simulink model "qpsk_srrc"  (R2012b)
settings: Solver=ode45  StartTime=0.0  StopTime=10.0  RelTol=1e-3
libraries: simulink x1
settings Model: Creator=Girish  LastModifiedBy=Girish

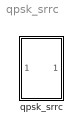
== system qpsk_srrc ==
  "qpsk_srrc " : Subsystem

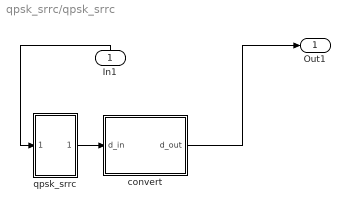
== system qpsk_srrc/qpsk_srrc  ==
  In1 : Inport
  convert : MATLAB Function  TreatAsAtomicUnit=on
  "qpsk_srrc " : Subsystem
  Out1 : Outport
  wires:
  convert/1(d_out) -> Out1/1
  "qpsk_srrc "/1(Out1) -> convert/1(d_in)
  In1/1 -> "qpsk_srrc "/1(In1)

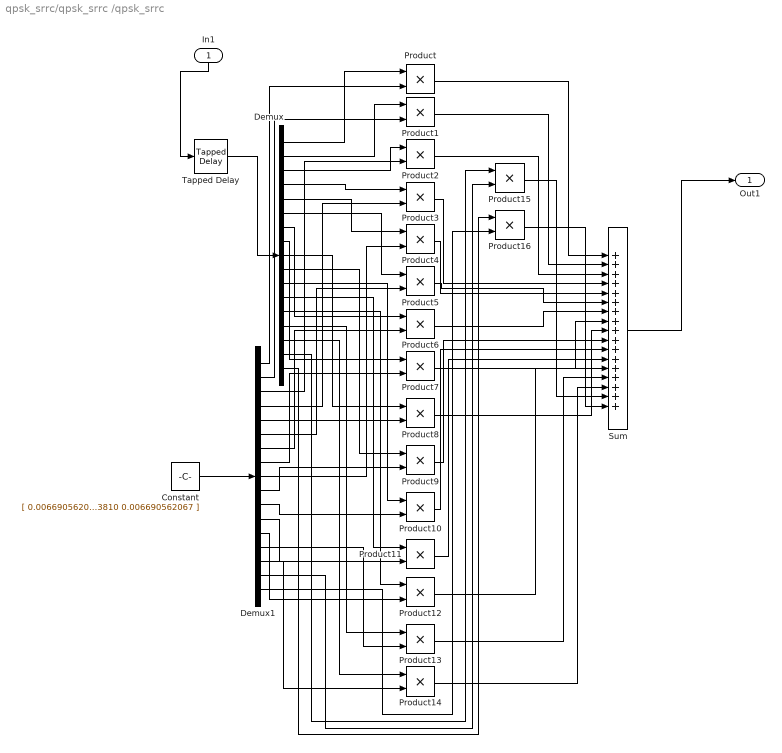
== system qpsk_srrc/qpsk_srrc /qpsk_srrc  ==
  In1 : Inport
  Constant : Constant  Value=|  OutDataTypeStr=fixdt(1,12,11)
      | [
      | 0.006690562067
      | -0.005768593810
      | -0.011827354519
      | 0.020586915021
      | 0.016726405168
      | -0.053692342207
      | -0.020253031546
      | 0.196043589067
      | 0.336822413190
      | 0.196043589067
      | -0.020253031546
      | -0.053692342207
      | 0.016726405168
      | 0.020586915021
      | -0.011827354519
      | -0.005768593810
      | 0.006690562067
      | ]
  Demux : Demux  Outputs=17
  Demux1 : Demux  Outputs=17
  Product{,1..16} (17 alike) : Product  RndMeth=Zero
  Sum : Sum  Inputs=|+|+|+|+|+|+|+|+|+|+|+|+|+|+|+|+|+
  Tapped Delay : simulink/Discrete/Tapped Delay  vinit=0.0  samptime=-1  NumDelays=17  DelayOrder=Newest  includeCurrent=off
  Out1 : Outport
  wires:
  In1/1 -> Tapped Delay/1
  Tapped Delay/1 -> Demux/1
  Demux/1 -> Product/1
  Demux/2 -> Product1/1
  Demux/3 -> Product2/1
  Demux/4 -> Product3/1
  Demux/5 -> Product4/1
  Demux/6 -> Product5/1
  Demux/7 -> Product6/1
  Demux/8 -> Product7/1
  Demux/9 -> Product8/1
  Demux/10 -> Product9/1
  Demux/11 -> Product10/1
  Demux/12 -> Product11/1
  Demux/13 -> Product12/1
  Demux/14 -> Product13/1
  Demux/15 -> Product14/1
  Demux/16 -> Product15/1
  Demux/17 -> Product16/1
  Constant/1 -> Demux1/1
  Demux1/1 -> Product/2
  Demux1/2 -> Product1/2
  Demux1/3 -> Product2/2
  Demux1/4 -> Product3/2
  Demux1/5 -> Product4/2
  Demux1/6 -> Product5/2
  Demux1/7 -> Product6/2
  Demux1/8 -> Product7/2
  Demux1/9 -> Product8/2
  Demux1/10 -> Product9/2
  Demux1/11 -> Product10/2
  Demux1/12 -> Product11/2
  Demux1/13 -> Product12/2
  Demux1/14 -> Product13/2
  Demux1/15 -> Product14/2
  Demux1/16 -> Product15/2
  Demux1/17 -> Product16/2
  Product/1 -> Sum/1
  Product1/1 -> Sum/2
  Product2/1 -> Sum/3
  Product3/1 -> Sum/4
  Product4/1 -> Sum/5
  Product5/1 -> Sum/6
  Product6/1 -> Sum/7
  Product7/1 -> Sum/8
  Product8/1 -> Sum/9
  Product9/1 -> Sum/10
  Product10/1 -> Sum/11
  Product11/1 -> Sum/12
  Product12/1 -> Sum/13
  Product13/1 -> Sum/14
  Product14/1 -> Sum/15
  Product15/1 -> Sum/16
  Product16/1 -> Sum/17
  Sum/1 -> Out1/1

== matlab function qpsk_srrc/qpsk_srrc /convert ==
  data: d_in input; d_out output
function d_out  = convert(d_in)

fm = hdlfimath;

d_out = fi(d_in, 1, 12, 11, fm);
